simulink model "Ejercicio_PID_manual"  (R2025b)
settings: Solver=VariableStepAuto  StartTime=0.0  StopTime=10.0  RelTol=1e-3
settings Model: Creator=Alexk  LastModifiedBy=Alexk

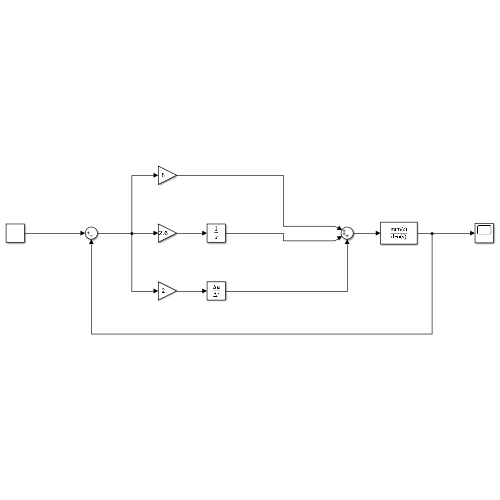
[thumbnail: Simulink's stored preview of the top-level diagram]
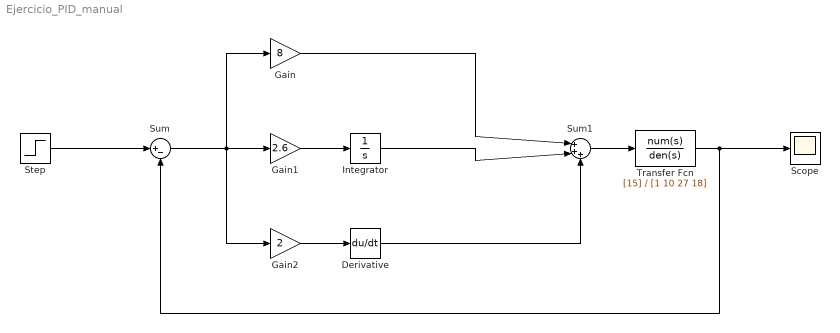
== system Ejercicio_PID_manual ==
  Derivative : Derivative
  Gain : Gain  Gain=8
  Gain1 : Gain  Gain=2.6
  Gain2 : Gain  Gain=2
  Integrator : Integrator
  Scope : Scope
      settings: ActiveDisplayYMinimum=-0.503767314000225  ActiveDisplayYMaximum=1.435041204872529
  Step : Step  Time=0  SampleTime=0
  Sum : Sum  Inputs=|+-
  Sum1 : Sum  Inputs=|+++
  Transfer Fcn : TransferFcn  Numerator=[15]  Denominator=[1 10 27 18]
  wires:
  Step/1 -> Sum/1
  Sum/1 -> Gain2/1, Gain1/1, Gain/1
  Gain1/1 -> Integrator/1
  Gain2/1 -> Derivative/1
  Gain/1 -> Sum1/1
  Integrator/1 -> Sum1/2
  Derivative/1 -> Sum1/3
  Sum1/1 -> Transfer Fcn/1
  Transfer Fcn/1 -> Scope/1, Sum/2
